simulink model "Model_SD_CIFB_k2"  (Simulink 10.0)
settings: Solver=VariableStepDiscrete  StartTime=0.0  StopTime=Tstop  RelTol=1e-3  EnableMultiTasking=on
values from neighbouring files (symbols this model uses):
  Amp = 10^(Av/20)*FS    (= 0.501187233627)    [run_Model_SD_CIFB_k2.m]
  fs = 2*BA*OSR    (= 2560000)    [run_Model_SD_CIFB_k2.m]
  OSR = 64    [run_Model_SD_CIFB_k2.m]
  ts = 1/fs    (= 3.90625e-07)    [run_Model_SD_CIFB_k2.m]
  win = 2*pi*fin    [run_Model_SD_CIFB_k2.m]
settings Model: Creator=cellierr  LastModifiedBy=corentin.pichat
settings DataIOCC: LimitDataPoints=on  SignalLoggingSaveFormat=ModelDataLogs
settings OptimizationCC: ExpressionDepthLimit=2147483647  InitFltsAndDblsToZero=on
settings DebuggingCC: SaveWithParameterizedLinksMsg=none  SolverPrmCheckMsg=warning  FcnCallInpInsideContextMsg=warning  StateNameClashWarn=warning
settings GRTTargetCC: TargetFcnLib=ansi_tfl_tmw.mat  GeneratePreprocessorConditionals=Disable all
settings ConfigComp: CovExternalEMLEnable=off  CovSFcnEnable=off

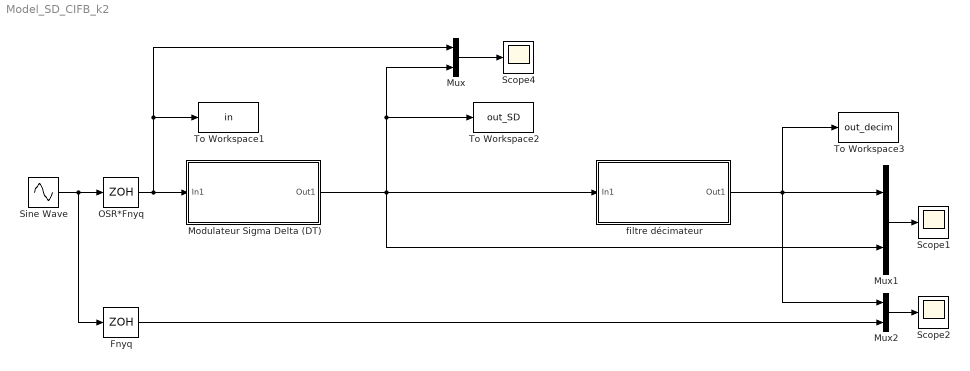
== system Model_SD_CIFB_k2 ==
  Fnyq : ZeroOrderHold  SampleTime=ts*OSR
  Modulateur Sigma Delta (DT) : Subsystem
  Mux : Mux  Inputs=2
  Mux1 : Mux  Inputs=2
  Mux2 : Mux  Inputs=2
  OSR*Fnyq : ZeroOrderHold  SampleTime=1/(fs)
  Scope1 : Scope
  Scope2 : Scope
  Scope4 : Scope
  Sine Wave : Sin  Amplitude=Amp  Frequency=win  SampleTime=0
  To Workspace1 : ToWorkspace  VariableName=in  SampleTime=-1
  To Workspace2 : ToWorkspace  VariableName=out_SD  SampleTime=-1
  To Workspace3 : ToWorkspace  VariableName=out_decim  SampleTime=ts
  filtre décimateur : Subsystem
  wires:
  Sine Wave/1 -> OSR*Fnyq/1, Fnyq/1
  OSR*Fnyq/1 -> Modulateur Sigma Delta (DT)/1(In1), Mux/1, To Workspace1/1
  Mux/1 -> Scope4/1
  Mux1/1 -> Scope1/1
  Fnyq/1 -> Mux2/2
  Mux2/1 -> Scope2/1
  Modulateur Sigma Delta (DT)/1(Out1) -> Mux1/2, filtre décimateur/1(In1), To Workspace2/1, Mux/2
  filtre décimateur/1(Out1) -> Mux2/1, To Workspace3/1, Mux1/1

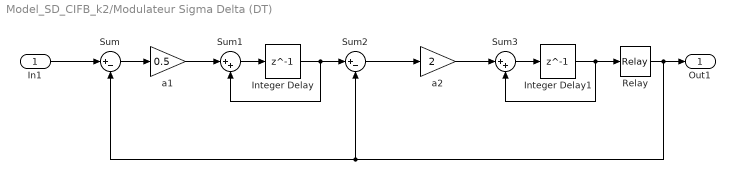
== system Model_SD_CIFB_k2/Modulateur Sigma Delta (DT) ==
  In1 : Inport
  Integer Delay : Delay  DelayLength=1
  Integer Delay1 : Delay  DelayLength=1
  Relay : Relay  OnSwitchValue=0  OffSwitchValue=0  OffOutputValue=-1
  Sum : Sum  Inputs=|+-
  Sum1 : Sum  Inputs=|++
  Sum2 : Sum  Inputs=|+-
  Sum3 : Sum  Inputs=|++
  a1 : Gain  Gain=0.5
  a2 : Gain  Gain=2
  Out1 : Outport
  wires:
  In1/1 -> Sum/1
  Sum/1 -> a1/1
  a1/1 -> Sum1/1
  Sum1/1 -> Integer Delay/1
  Integer Delay/1 -> Sum2/1, Sum1/2
  Sum2/1 -> a2/1
  a2/1 -> Sum3/1
  Sum3/1 -> Integer Delay1/1
  Integer Delay1/1 -> Relay/1, Sum3/2
  Relay/1 -> Sum2/2, Sum/2, Out1/1

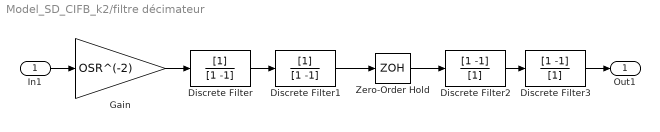
== system Model_SD_CIFB_k2/filtre décimateur ==
  In1 : Inport
  Discrete Filter : DiscreteFilter  Denominator=[1 -1]
  Discrete Filter1 : DiscreteFilter  Denominator=[1 -1]
  Discrete Filter2 : DiscreteFilter  Numerator=[1 -1]  Denominator=[1]  SampleTime=ts*OSR
  Discrete Filter3 : DiscreteFilter  Numerator=[1 -1]  Denominator=[1]  SampleTime=ts*OSR
  Gain : Gain  Gain=OSR^(-2)  SaturateOnIntegerOverflow=on  OutDataTypeStr=Inherit: Same as input  ParamDataTypeStr=Inherit: Same as input
  Zero-Order Hold : ZeroOrderHold  SampleTime=ts*OSR
  Out1 : Outport
  wires:
  In1/1 -> Gain/1
  Discrete Filter3/1 -> Out1/1
  Gain/1 -> Discrete Filter/1
  Discrete Filter/1 -> Discrete Filter1/1
  Discrete Filter2/1 -> Discrete Filter3/1
  Discrete Filter1/1 -> Zero-Order Hold/1
  Zero-Order Hold/1 -> Discrete Filter2/1
